simulink model "Sat_Nonliner_N_P_2"  (R2024a)
settings: Solver=ode45  StartTime=0.0  StopTime=20000  RelTol=1e-3  EnableMultiTasking=on
model workspace (MAT data in the model file):
  Q_fenzi = [2.841 -4.406 1.749]
values from neighbouring files (symbols this model uses):
  sat_alpha = sat_alpha_set_3_main(sat_alpha_i)    [SAT_MAIN.m]    (also in Sat_Model_G.m = 5; Sat_Model_N_P.m = sat_alpha_set(sat_alpha_i); model_sat_n_p.m = sat_alpha_1)
settings Model: Creator=75499  LastModifiedBy=xthinking
settings SolverCC: AlgebraicLoopSolver=TrustRegion
settings DataIOCC: LimitDataPoints=on  SaveFormat=Array  SignalLoggingSaveFormat=ModelDataLogs  ReturnWorkspaceOutputs=off
settings OptimizationCC: ExpressionDepthLimit=2147483647  LifeSpan=inf
settings DebuggingCC: UnderspecifiedInitializationDetection=Classic  MergeDetectMultiDrivingBlocksExec=none  SolverPrmCheckMsg=warning  FcnCallInpInsideContextMsg=warning  UnconnectedInputMsg=warning  UnconnectedOutputMsg=warning  UnconnectedLineMsg=warning  StateNameClashWarn=warning  SFUnexpectedBacktrackingDiag=warning  SFNoUnconditionalDefaultTransitionDiag=warning  SFExecutionAtInitializationDiag=none  ArithmeticOperatorsInVariantConditions=warning
settings HardwareCC: ProdBitPerPointer=32  ProdBitPerSizeT=32  ProdBitPerPtrDiffT=32  ProdLargestAtomicFloat=None  ProdIntDivRoundTo=Undefined  ProdEndianess=Unspecified  ProdWordSize=32  ProdHWDeviceType=32-bit Generic
settings ModelReferenceCC: EnableRefExpFcnMdlSchedulingChecks=on  PropagateSignalLabelsOutOfModel=off
settings SFSimCC: SimUseLocalCustomCode=off  CustomCodeUndefinedFunction=UseInterfaceOnly
settings RTWCC: RTWUseLocalCustomCode=off  GPUComputeCapability=3.5
settings CodeAppCC: StateflowObjectComments=on
settings GRTTargetCC: TargetLangStandard=C89/C90 (ANSI)
settings ConfigComp: CovMetricSettings=dw  CovSaveCumulativeToWorkspaceVar=on  CovSaveSingleToWorkspaceVar=on  CovExternalEMLEnable=off

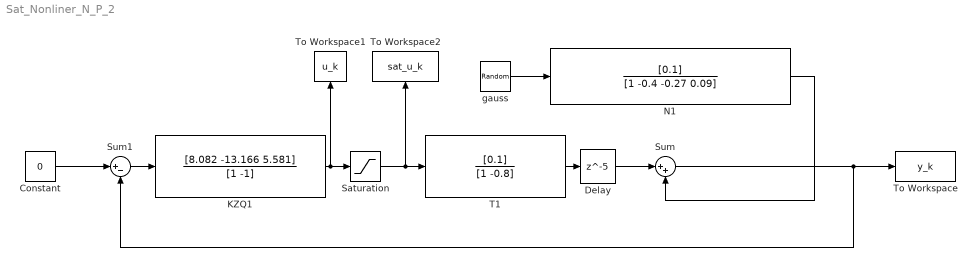
== system Sat_Nonliner_N_P_2 ==
  Constant : Constant  Value=0
  Delay : Delay  DelayLength=5
  KZQ1 : DiscreteFilter  Numerator=[8.082 -13.166 5.581]  Denominator=[1 -1]
  N1 : DiscreteFilter  Numerator=[0.1]  Denominator=[1 -0.4 -0.27 0.09]
  Saturation : Saturate  UpperLimit=sat_alpha  LowerLimit=-sat_alpha  ZeroCross=off
  Sum : Sum  Inputs=|++
  Sum1 : Sum  Inputs=|+-
  T1 : DiscreteFilter  Numerator=[0.1]  Denominator=[1 -0.8]
  To Workspace : ToWorkspace  VariableName=y_k  SampleTime=-1
  To Workspace1 : ToWorkspace  VariableName=u_k  SampleTime=-1
  To Workspace2 : ToWorkspace  VariableName=sat_u_k  SampleTime=-1
  gauss : RandomNumber  SampleTime=0.1
  wires:
  gauss/1 -> N1/1
  T1/1 -> Delay/1
  Delay/1 -> Sum/1
  N1/1 -> Sum/2
  Sum/1 -> To Workspace/1, Sum1/2
  Constant/1 -> Sum1/1
  Sum1/1 -> KZQ1/1
  Saturation/1 -> T1/1, To Workspace2/1
  KZQ1/1 -> Saturation/1, To Workspace1/1
